simulink model "Lead_Lag_Compensator"  (R2018a)
settings: Solver=VariableStepAuto  StartTime=0.0  StopTime=10.0  RelTol=1e-3
settings Model: Creator=David  LastModifiedBy=David

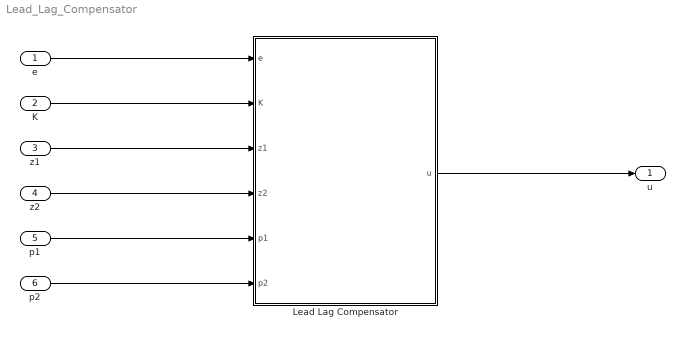
== system Lead_Lag_Compensator ==
  e : Inport
  K : Inport  Port=2
  z1 : Inport  Port=3
  z2 : Inport  Port=4
  p1 : Inport  Port=5
  p2 : Inport  Port=6
  Lead Lag Compensator : Subsystem
      mask Display:
      | disp('K(s-z1)(s-z2)/(s-p1)(s-p2)')
      | 
      | port_label('input', 1, 'e')
      | port_label('input', 2, 'K')
      | port_label('input', 3, 'z1')
      | port_label('input', 4, 'z2')
      | port_label('input', 5, 'p1')
      | port_label('input', 6, 'p2')
      | 
      | port_label('output', 1, 'u')
  u : Outport
  wires:
  e/1 -> Lead Lag Compensator/1(e)
  K/1 -> Lead Lag Compensator/2(K)
  z1/1 -> Lead Lag Compensator/3(z1)
  z2/1 -> Lead Lag Compensator/4(z2)
  p1/1 -> Lead Lag Compensator/5(p1)
  p2/1 -> Lead Lag Compensator/6(p2)
  Lead Lag Compensator/1(u) -> u/1

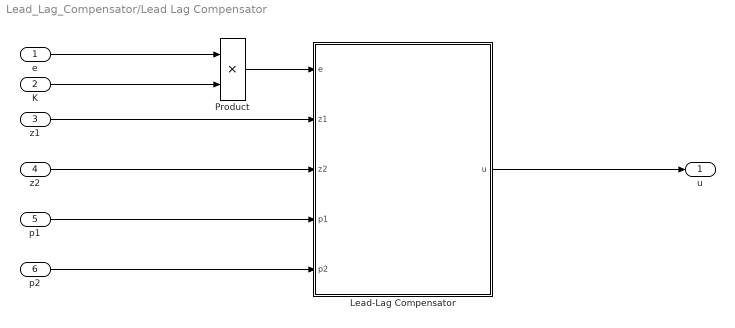
== system Lead_Lag_Compensator/Lead Lag Compensator ==
  e : Inport
  K : Inport  Port=2
  z1 : Inport  Port=3
  z2 : Inport  Port=4
  p1 : Inport  Port=5
  p2 : Inport  Port=6
  Lead-Lag Compensator : Subsystem
      mask Display:
      | disp('(s-z1)(s-z2)/(s-p1)(s-p2)')
      | 
      | port_label('input', 1, 'e')
      | port_label('input', 2, 'z1')
      | port_label('input', 3, 'z2')
      | port_label('input', 4, 'p1')
      | port_label('input', 5, 'p2')
      | 
      | port_label('output', 1, 'u')
  Product : Product
  u : Outport
  wires:
  e/1 -> Product/1
  z2/1 -> Lead-Lag Compensator/3(z2)
  Product/1 -> Lead-Lag Compensator/1(e)
  Lead-Lag Compensator/1(u) -> u/1
  p2/1 -> Lead-Lag Compensator/5(p2)
  p1/1 -> Lead-Lag Compensator/4(p1)
  z1/1 -> Lead-Lag Compensator/2(z1)
  K/1 -> Product/2

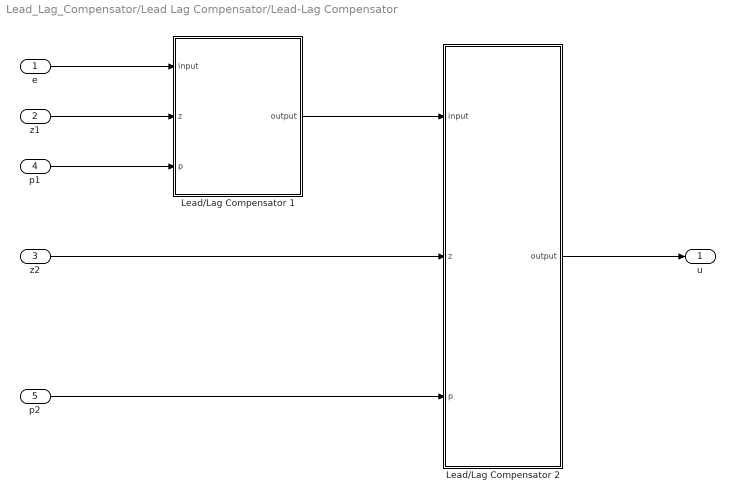
== system Lead_Lag_Compensator/Lead Lag Compensator/Lead-Lag Compensator ==
  e : Inport
  z1 : Inport  Port=2
  z2 : Inport  Port=3
  p1 : Inport  Port=4
  p2 : Inport  Port=5
  Lead/Lag Compensator 1 : Subsystem
      mask Display:
      | disp('s-z/s-p')
      | 
      | port_label('input', 1, 'e')
      | port_label('input', 2, 'z')
      | port_label('input', 3, 'p')
      | 
      | port_label('output', 1, 'y')
  Lead/Lag Compensator 2 : Subsystem
      mask Display:
      | disp('s-z/s-p')
      | 
      | port_label('input', 1, 'e')
      | port_label('input', 2, 'z')
      | port_label('input', 3, 'p')
      | 
      | port_label('output', 1, 'y')
  u : Outport
  wires:
  p1/1 -> Lead/Lag Compensator 1/3(p)
  e/1 -> Lead/Lag Compensator 1/1(input)
  p2/1 -> Lead/Lag Compensator 2/3(p)
  z2/1 -> Lead/Lag Compensator 2/2(z)
  z1/1 -> Lead/Lag Compensator 1/2(z)
  Lead/Lag Compensator 2/1(output) -> u/1
  Lead/Lag Compensator 1/1(output) -> Lead/Lag Compensator 2/1(input)

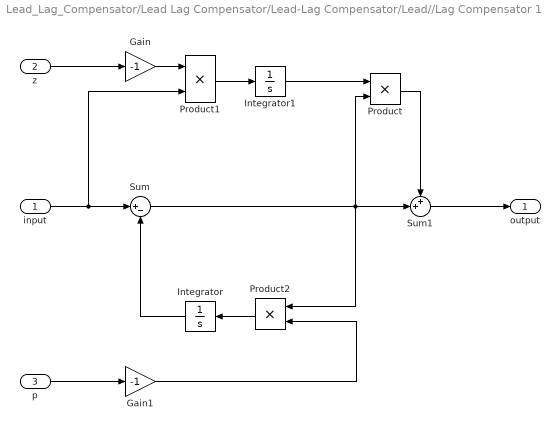
== system Lead_Lag_Compensator/Lead Lag Compensator/Lead-Lag Compensator/Lead//Lag Compensator 1 ==
  input : Inport
  z : Inport  Port=2
  p : Inport  Port=3
  Gain : Gain  Gain=-1
  Gain1 : Gain  Gain=-1
  Integrator : Integrator
  Integrator1 : Integrator
  Product : Product
  Product1 : Product
  Product2 : Product
  Sum : Sum  Inputs=|+-
  Sum1 : Sum  Inputs=++|
  output : Outport
  wires:
  Integrator/1 -> Sum/2
  Sum/1 -> Product2/1, Product/2, Sum1/2
  Product2/1 -> Integrator/1
  Integrator1/1 -> Product/1
  Gain/1 -> Product1/1
  p/1 -> Gain1/1
  Gain1/1 -> Product2/2
  Product/1 -> Sum1/1
  input/1 -> Product1/2, Sum/1
  Sum1/1 -> output/1
  Product1/1 -> Integrator1/1
  z/1 -> Gain/1

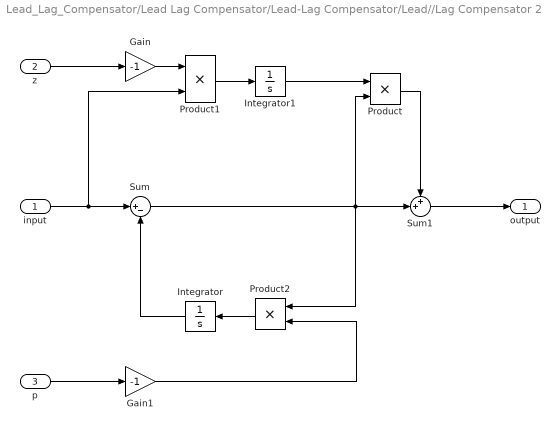
== system Lead_Lag_Compensator/Lead Lag Compensator/Lead-Lag Compensator/Lead//Lag Compensator 2 ==
  input : Inport
  z : Inport  Port=2
  p : Inport  Port=3
  Gain : Gain  Gain=-1
  Gain1 : Gain  Gain=-1
  Integrator : Integrator
  Integrator1 : Integrator
  Product : Product
  Product1 : Product
  Product2 : Product
  Sum : Sum  Inputs=|+-
  Sum1 : Sum  Inputs=++|
  output : Outport
  wires:
  Integrator/1 -> Sum/2
  Sum/1 -> Product2/1, Product/2, Sum1/2
  Product2/1 -> Integrator/1
  Integrator1/1 -> Product/1
  Gain/1 -> Product1/1
  p/1 -> Gain1/1
  Gain1/1 -> Product2/2
  Product/1 -> Sum1/1
  input/1 -> Product1/2, Sum/1
  Sum1/1 -> output/1
  Product1/1 -> Integrator1/1
  z/1 -> Gain/1
